simulink model "guidepath_system"  (R2016a)
settings: Solver=VariableStepAuto  StartTime=0.0  StopTime=30  RelTol=1e-3
libraries: simulink x1
settings Model: Creator=wesleyfinck  LastModifiedBy=wesleyfinck

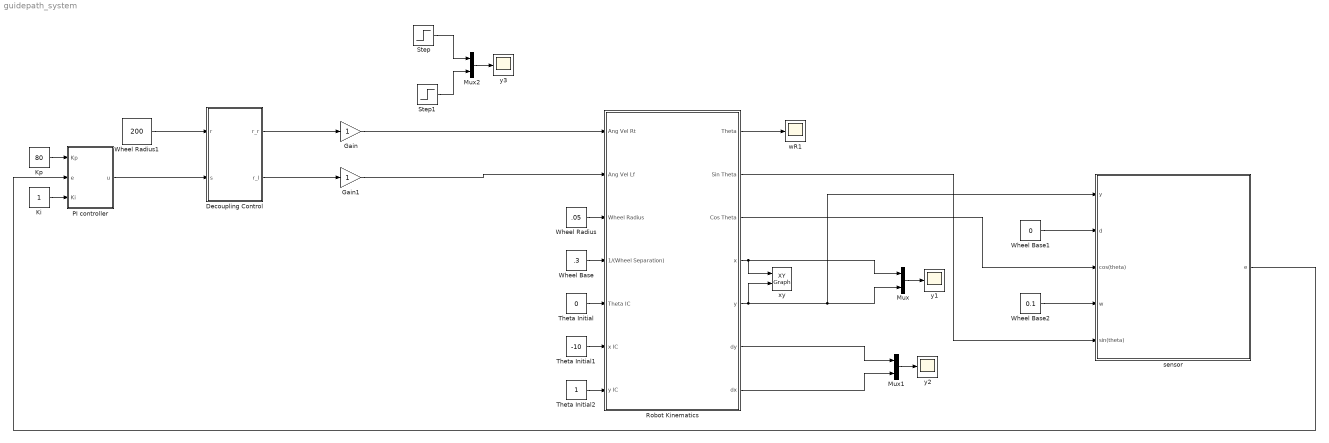
== system guidepath_system ==
  Decoupling Control : Subsystem
  Gain : Gain
  Gain1 : Gain
  Ki : Constant
  Kp : Constant  Value=80
  Mux : Mux  Inputs=2
  Mux1 : Mux  Inputs=2
  Mux2 : Mux  Inputs=2
  PI controller : Subsystem
  Robot Kinematics : Subsystem
  Step : Step  Time=10  Before=50  After=-20  SampleTime=0
  Step1 : Step  Time=10  Before=50  After=-20  SampleTime=0
  Theta Initial : Constant  Value=0  VectorParams1D=off  OutDataTypeStr=double
  Theta Initial1 : Constant  Value=-10  VectorParams1D=off  OutDataTypeStr=double
  Theta Initial2 : Constant  VectorParams1D=off  OutDataTypeStr=double
  Wheel Base : Constant  Value=.3
  Wheel Base1 : Constant  Value=0
  Wheel Base2 : Constant  Value=0.1
  Wheel Radius : Constant  Value=.05
  Wheel Radius1 : Constant  Value=200
  sensor : Subsystem
  wR1 : Scope
  xy : simulink/Sinks/XY Graph  xmin=-20  xmax=300  ymin=-5  ymax=5  st=-1
  y1 : Scope
  y2 : Scope
  y3 : Scope
  wires:
  Wheel Radius/1 -> Robot Kinematics/3(Wheel Radius)
  Wheel Base/1 -> Robot Kinematics/4(1/(Wheel Separation))
  Theta Initial/1 -> Robot Kinematics/5(Theta IC)
  Robot Kinematics/5(y) -> xy/2, sensor/1(y), Mux/2
  Robot Kinematics/4(x) -> xy/1, Mux/1
  Step1/1 -> Mux2/2
  Step/1 -> Mux2/1
  Robot Kinematics/7(dx) -> Mux1/2
  Robot Kinematics/6(dy) -> Mux1/1
  Mux1/1 -> y2/1
  Robot Kinematics/1(Theta) -> wR1/1
  Mux/1 -> y1/1
  Mux2/1 -> y3/1
  Decoupling Control/1(r_r) -> Gain/1
  Decoupling Control/2("r_l ") -> Gain1/1
  Wheel Radius1/1 -> Decoupling Control/1(r)
  Wheel Base1/1 -> sensor/2(d)
  Robot Kinematics/3(Cos Theta) -> sensor/3(cos(theta))
  Robot Kinematics/2(Sin Theta) -> sensor/5(sin(theta))
  Wheel Base2/1 -> sensor/4(w)
  Theta Initial2/1 -> Robot Kinematics/7(y IC)
  Theta Initial1/1 -> Robot Kinematics/6(x IC)
  Gain/1 -> Robot Kinematics/1(Ang Vel Rt)
  Gain1/1 -> Robot Kinematics/2(Ang Vel Lf)
  Kp/1 -> PI controller/1(Kp)
  sensor/1(e) -> PI controller/2(e)
  Ki/1 -> PI controller/3(Ki)
  PI controller/1(u) -> Decoupling Control/2(s)

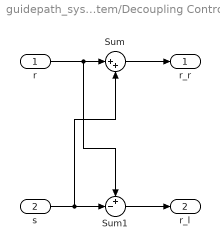
== system guidepath_system/Decoupling Control ==
  r : Inport
  s : Inport  Port=2
  Sum : Sum  Inputs=|++
  Sum1 : Sum  Inputs=+-|
  r_r : Outport
  "r_l " : Outport  Port=2
  wires:
  Sum1/1 -> "r_l "/1
  s/1 -> Sum/2, Sum1/2
  r/1 -> Sum1/1, Sum/1
  Sum/1 -> r_r/1

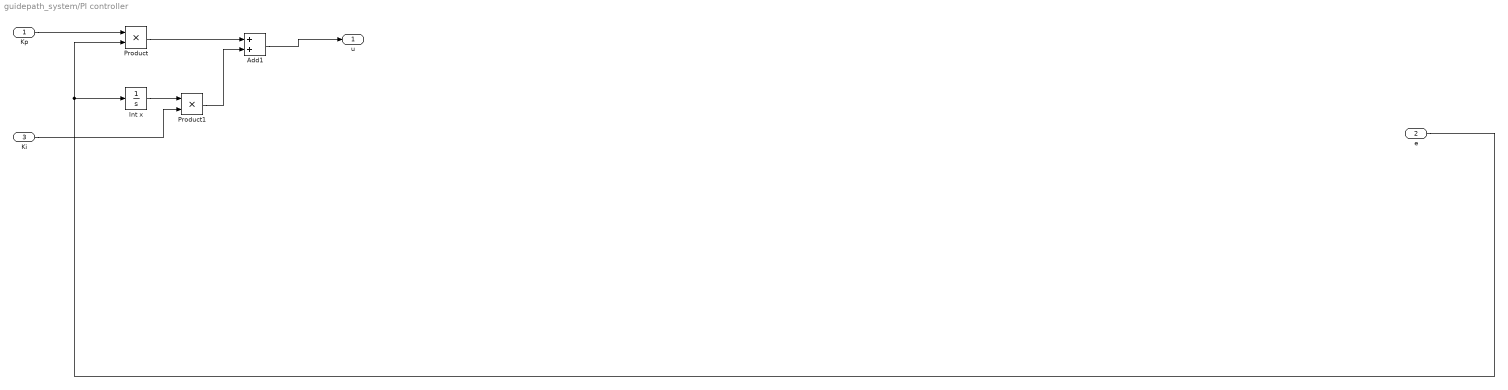
== system guidepath_system/PI controller ==
  Kp : Inport
  e : Inport  Port=2
  Ki : Inport  Port=3
  Add1 : Sum
  Int x : Integrator
  Product : Product
  Product1 : Product
  u : Outport
  wires:
  e/1 -> Int x/1, Product/2
  Add1/1 -> u/1
  Kp/1 -> Product/1
  Ki/1 -> Product1/2
  Product1/1 -> Add1/2
  Product/1 -> Add1/1
  Int x/1 -> Product1/1

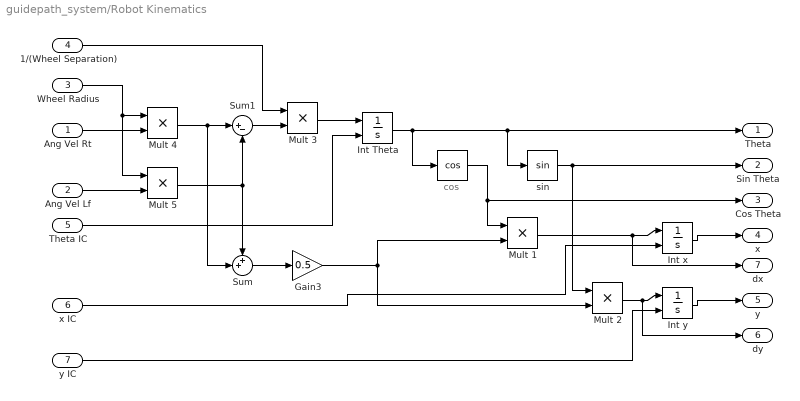
== system guidepath_system/Robot Kinematics ==
  note: cos
  Ang Vel Rt : Inport
  Ang Vel Lf : Inport  Port=2
  Wheel Radius : Inport  Port=3
  1/(Wheel Separation) : Inport  Port=4
  Theta IC : Inport  Port=5
  x IC : Inport  Port=6
  y IC : Inport  Port=7
  " " : Trigonometry  Operator=cos
  Gain3 : Gain  Gain=0.5
  Int Theta : Integrator  InitialConditionSource=external  InitialCondition=1  ZeroCross=off
  Int x : Integrator  InitialConditionSource=external
  Int y : Integrator  InitialConditionSource=external
  Mult {1..5} (5 alike) : Product  RndMeth=Zero
  Sum : Sum  Inputs=++|
  Sum1 : Sum  Inputs=|+-
  sin : Trigonometry
  Theta : Outport
  Sin Theta : Outport  Port=2
  Cos Theta : Outport  Port=3
  x : Outport  Port=4
  y : Outport  Port=5
  dy : Outport  Port=6
  dx : Outport  Port=7
  wires:
  Mult 4/1 -> Sum1/1, Sum/2
  Mult 5/1 -> Sum1/2, Sum/1
  Sum1/1 -> Mult 3/2
  Sum/1 -> Gain3/1
  Int Theta/1 -> " "/1, sin/1, Theta/1
  Gain3/1 -> Mult 1/2, Mult 2/2
  " "/1 -> Mult 1/1, Cos Theta/1
  Mult 1/1 -> Int x/1, dx/1
  Mult 2/1 -> Int y/1, dy/1
  sin/1 -> Mult 2/1, Sin Theta/1
  Int x/1 -> x/1
  Int y/1 -> y/1
  Mult 3/1 -> Int Theta/1
  Ang Vel Lf/1 -> Mult 5/2
  Ang Vel Rt/1 -> Mult 4/2
  Wheel Radius/1 -> Mult 4/1, Mult 5/1
  1/(Wheel Separation)/1 -> Mult 3/1
  Theta IC/1 -> Int Theta/2
  x IC/1 -> Int x/2
  y IC/1 -> Int y/2

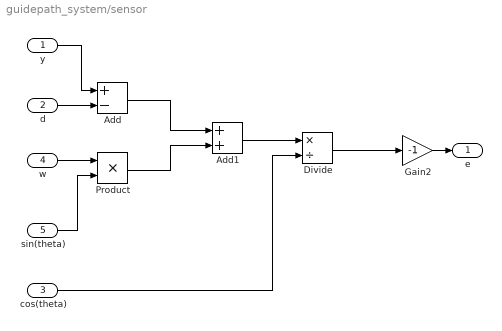
== system guidepath_system/sensor ==
  y : Inport
  d : Inport  Port=2
  cos(theta) : Inport  Port=3
  w : Inport  Port=4
  sin(theta) : Inport  Port=5
  Add : Sum  Inputs=+-
  Add1 : Sum
  Divide : Product  Inputs=*/
  Gain2 : Gain  Gain=-1
  Product : Product
  e : Outport
  wires:
  Divide/1 -> Gain2/1
  cos(theta)/1 -> Divide/2
  Add/1 -> Add1/1
  Gain2/1 -> e/1
  Add1/1 -> Divide/1
  d/1 -> Add/2
  Product/1 -> Add1/2
  sin(theta)/1 -> Product/2
  w/1 -> Product/1
  y/1 -> Add/1
